simulink model "motor_model_8__um"  (R2020a)
settings: Solver=VariableStepAuto  StartTime=0.0  StopTime=7  RelTol=1e-7
model workspace (MAT data in the model file):
  A01 = 0.209333333333
  A1 = 0.035
  A2 = 0.21
  Ai = 0.348888888889
  Fi = 3.14
  K = 1500
  Km = 33.68
  Kn = 8.33
  Mn = 0.08
  T1 = 0.05
  T2 = 0.0005
  Te = 0.0004
  Tm = 0.29
  Tpwm = 6.25e-05
  U = 100
  dangle = 0.000383
  omega1 = 6.28
  omega2 = 1.005
  target_ = 3.14
libraries: simulink x1
settings Model: Creator=Sainquake  LastModifiedBy=Sainquake
settings DataIOCC: ReturnWorkspaceOutputs=off
settings DebuggingCC: ArithmeticOperatorsInVariantConditions=warning
settings SFSimCC: CustomCodeUndefinedFunction=UseInterfaceOnly

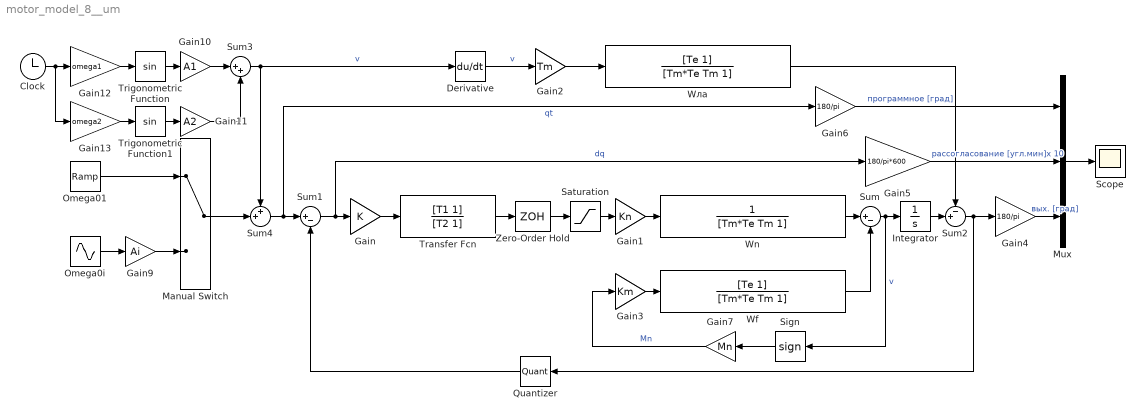
== system motor_model_8__um ==
  Clock : Clock
  Derivative : Derivative
  Gain : Gain  Gain=K
  Gain1 : Gain  Gain=Kn
  Gain10 : Gain  Gain=A1
  Gain11 : Gain  Gain=A2
  Gain12 : Gain  Gain=omega1
  Gain13 : Gain  Gain=omega2
  Gain2 : Gain  Gain=Tm
  Gain3 : Gain  Gain=Km
  Gain4 : Gain  Gain=180/pi
  Gain5 : Gain  Gain=180/pi*600
  Gain6 : Gain  Gain=180/pi
  Gain7 : Gain  Gain=Mn
  Gain9 : Gain  Gain=Ai
  Integrator : Integrator
  Manual Switch : ManualSwitch
  Mux : Mux  Inputs=3
  Omega01 : simulink/Sources/Ramp  slope=12/180*3.14  start=0  InitialOutput=0
  Omega0i : Sin  Frequency=Fi  SampleTime=0
  Quantizer : Quantizer  QuantizationInterval=dangle/4
  Saturation : Saturate  UpperLimit=U  LowerLimit=-U
  Scope : Scope
  Sign : Signum  ZeroCross=off
  Sum : Sum  Inputs=|+-
  Sum1 : Sum  Inputs=|+-
  Sum2 : Sum  Inputs=-+|
  Sum3 : Sum  Inputs=|++
  Sum4 : Sum  Inputs=++|
  Transfer Fcn : TransferFcn  Numerator=[T1 1]  Denominator=[T2 1]
  Trigonometric Function : Trigonometry
  Trigonometric Function1 : Trigonometry
  Wf : TransferFcn  Numerator=[Te 1]  Denominator=[Tm*Te Tm 1]
  "Wn " : TransferFcn  Denominator=[Tm*Te Tm 1]
  Wла : TransferFcn  Numerator=[Te 1]  Denominator=[Tm*Te Tm 1]
  Zero-Order Hold : ZeroOrderHold  SampleTime=Tpwm
  wires:
  Sum1/1 -> Gain5/1, Gain/1  "dq"
  Sum4/1 -> Gain6/1, Sum1/1  "qt"
  Sum2/1 -> Quantizer/1, Gain4/1
  Gain7/1 -> Gain3/1  "Mn"
  Sum3/1 -> Derivative/1, Sum4/1  "v"
  Gain/1 -> Transfer Fcn/1
  Integrator/1 -> Sum2/2
  "Wn "/1 -> Sum/1
  Wла/1 -> Sum2/1
  Wf/1 -> Sum/2
  Gain1/1 -> "Wn "/1
  Gain2/1 -> Wла/1
  Gain3/1 -> Wf/1
  Gain4/1 -> Mux/3  "вых. [град]"
  Gain5/1 -> Mux/2  "рассогласование [угл.мин]x 10"
  Gain6/1 -> Mux/1  "программное [град]"
  Mux/1 -> Scope/1
  Quantizer/1 -> Sum1/2
  Transfer Fcn/1 -> Zero-Order Hold/1
  Omega0i/1 -> Gain9/1
  Gain12/1 -> Trigonometric Function/1
  Trigonometric Function/1 -> Gain10/1
  Clock/1 -> Gain12/1, Gain13/1
  Gain11/1 -> Sum3/2
  Trigonometric Function1/1 -> Gain11/1
  Gain13/1 -> Trigonometric Function1/1
  Gain10/1 -> Sum3/1
  Sign/1 -> Gain7/1
  Sum/1 -> Sign/1, Integrator/1  "v"
  Derivative/1 -> Gain2/1  "v"
  Manual Switch/1 -> Sum4/2
  Gain9/1 -> Manual Switch/2
  Omega01/1 -> Manual Switch/1
  Zero-Order Hold/1 -> Saturation/1
  Saturation/1 -> Gain1/1
